simulink model "SustituirTerminoIEnC3"  (R2023a)
settings: Solver=FixedStepDiscrete  StartTime=0.0  StopTime=7430  FixedStep=Delta  RelTol=1e-3
values from neighbouring files (symbols this model uses):
  C2Ini = 1.6    [MassTransferModelData.m]
  C3Ini = 0    [MassTransferModelData.m]
  C4Ini = 0    [MassTransferModelData.m]
  C5Ini = 1.6    [MassTransferModelData.m]
  Delta = 5    [MassTransferModelData.m]
  F = 96485    [MassTransferModelData.m]
  NCells = 120    [MassTransferModelData.m]
  VCell = 0.4968    [MassTransferModelData.m]
  VTank = 500    [MassTransferModelData.m]
  z = 1    [MassTransferModelData.m]
undefined symbols (not defined in the file or in its folder): DiscIntNeverNeededParam
settings Model: Creator=801896  LastModifiedBy=801896

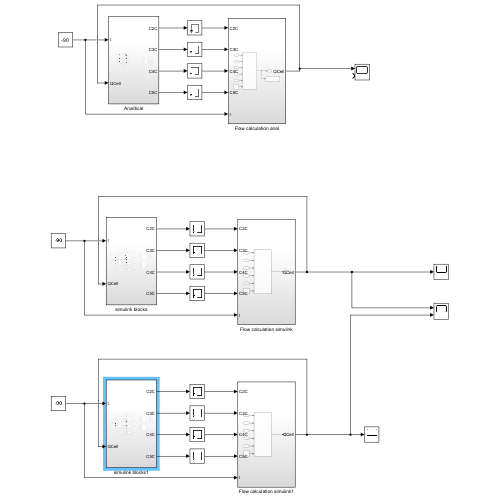
[thumbnail: Simulink's stored preview of the top-level diagram]
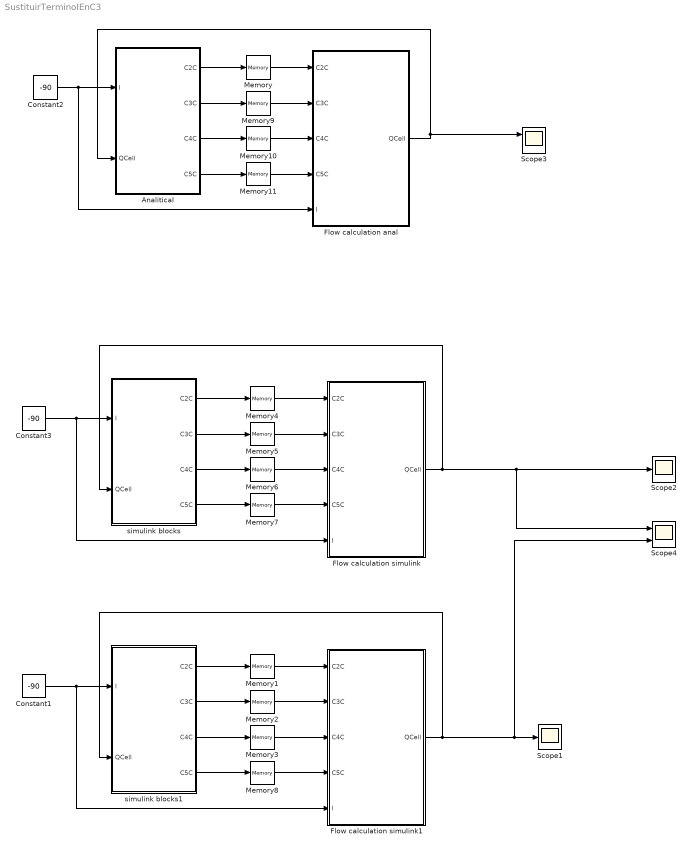
== system SustituirTerminoIEnC3 ==
  Analitical : Subsystem
  Constant1 : Constant  Value=-90
  Constant2 : Constant  Value=-90
  Constant3 : Constant  Value=-90
  Flow calculation anal : Subsystem
  Flow calculation simulink : Subsystem
  Flow calculation simulink1 : Subsystem
  Memory : Memory  InitialCondition=C2Ini
  Memory1 : Memory  InitialCondition=C2Ini
  Memory10 : Memory  InitialCondition=C4Ini
  Memory11 : Memory  InitialCondition=C5Ini
  Memory2 : Memory  InitialCondition=C3Ini
  Memory3 : Memory  InitialCondition=C4Ini
  Memory4 : Memory  InitialCondition=C2Ini
  Memory5 : Memory  InitialCondition=C3Ini
  Memory6 : Memory  InitialCondition=C4Ini
  Memory7 : Memory  InitialCondition=C5Ini
  Memory8 : Memory  InitialCondition=C5Ini
  Memory9 : Memory  InitialCondition=C3Ini
  Scope1 : Scope
  Scope2 : Scope
  Scope3 : Scope  NumInputPorts=2
  Scope4 : Scope  NumInputPorts=2
  simulink blocks : Subsystem
  simulink blocks1 : Subsystem
  wires:
  simulink blocks/3(C4C) -> Memory6/1
  Constant3/1 -> Flow calculation simulink/5(I), simulink blocks/1(I)
  Memory4/1 -> Flow calculation simulink/1(C2C)
  simulink blocks/1(C2C) -> Memory4/1
  Memory6/1 -> Flow calculation simulink/3(C4C)
  Memory7/1 -> Flow calculation simulink/4(C5C)
  simulink blocks/2(C3C) -> Memory5/1
  Memory5/1 -> Flow calculation simulink/2(C3C)
  simulink blocks/4(C5C) -> Memory7/1
  Flow calculation simulink/1(QCell) -> Scope4/1, Scope2/1, simulink blocks/2(QCell)
  Flow calculation simulink1/1(QCell) -> simulink blocks1/2(QCell), Scope4/2, Scope1/1
  simulink blocks1/4(C5C) -> Memory8/1
  Memory2/1 -> Flow calculation simulink1/2(C3C)
  simulink blocks1/2(C3C) -> Memory2/1
  Memory8/1 -> Flow calculation simulink1/4(C5C)
  Memory3/1 -> Flow calculation simulink1/3(C4C)
  simulink blocks1/1(C2C) -> Memory1/1
  Memory1/1 -> Flow calculation simulink1/1(C2C)
  Constant1/1 -> simulink blocks1/1(I), Flow calculation simulink1/5(I)
  simulink blocks1/3(C4C) -> Memory3/1
  Memory/1 -> Flow calculation anal/1(C2C)
  Analitical/1(C2C) -> Memory/1
  Analitical/4(C5C) -> Memory11/1
  Memory9/1 -> Flow calculation anal/2(C3C)
  Memory10/1 -> Flow calculation anal/3(C4C)
  Analitical/3(C4C) -> Memory10/1
  Memory11/1 -> Flow calculation anal/4(C5C)
  Analitical/2(C3C) -> Memory9/1
  Constant2/1 -> Flow calculation anal/5(I), Analitical/1(I)
  Flow calculation anal/1(QCell) -> Analitical/2(QCell), Scope3/1

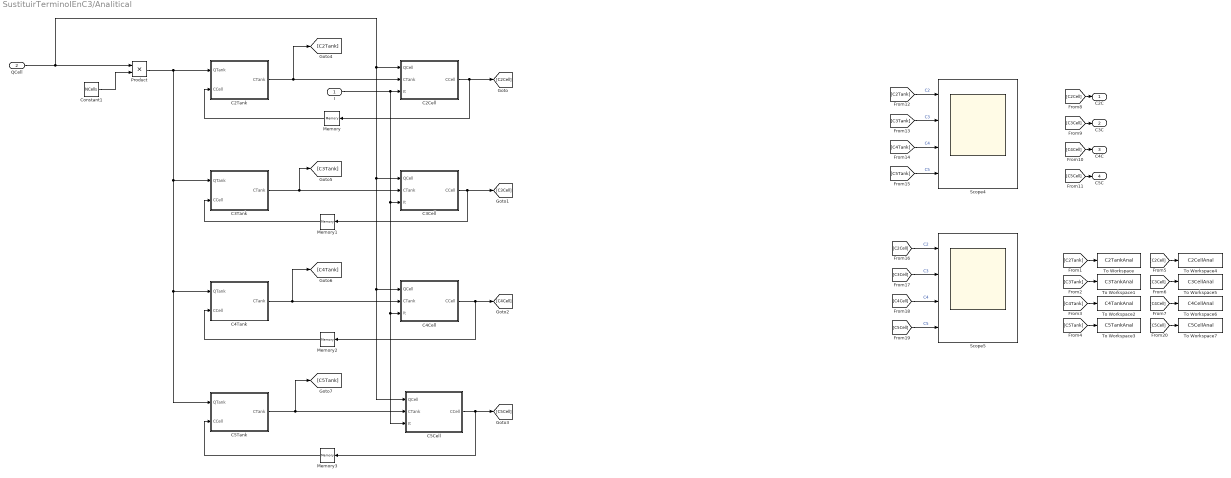
== system SustituirTerminoIEnC3/Analitical ==
  I : Inport
  QCell : Inport  Port=2
  C2Cell : Subsystem
  C2Tank : Subsystem
  C3Cell : Subsystem
  C3Tank : Subsystem
  C4Cell : Subsystem
  C4Tank : Subsystem
  C5Cell : Subsystem
  C5Tank : Subsystem
  Constant1 : Constant  Value=NCells
  Memory : Memory  InitialCondition=C2Ini
  Memory1 : Memory  InitialCondition=C3Ini
  Memory2 : Memory  InitialCondition=C4Ini
  Memory3 : Memory  InitialCondition=C5Ini
  Product : Product
  Scope4 : Scope  NumInputPorts=4
  Scope5 : Scope  NumInputPorts=4
  To Workspace : ToWorkspace  VariableName=C2TankAnal  SaveFormat=Timeseries  SampleTime=-1
  To Workspace1 : ToWorkspace  VariableName=C3TankAnal  SaveFormat=Timeseries  SampleTime=-1
  To Workspace2 : ToWorkspace  VariableName=C4TankAnal  SaveFormat=Timeseries  SampleTime=-1
  To Workspace3 : ToWorkspace  VariableName=C5TankAnal  SaveFormat=Timeseries  SampleTime=-1
  To Workspace4 : ToWorkspace  VariableName=C2CellAnal  SaveFormat=Timeseries  SampleTime=-1
  To Workspace5 : ToWorkspace  VariableName=C3CellAnal  SaveFormat=Timeseries  SampleTime=-1
  To Workspace6 : ToWorkspace  VariableName=C4CellAnal  SaveFormat=Timeseries  SampleTime=-1
  To Workspace7 : ToWorkspace  VariableName=C5CellAnal  SaveFormat=Timeseries  SampleTime=-1
  C2C : Outport
  C3C : Outport  Port=2
  C4C : Outport  Port=3
  C5C : Outport  Port=4
  wires:
  [C5Cell] -> C5C/1
  [C3Cell] -> C3C/1
  [C2Cell] -> C2C/1
  [C4Cell] -> C4C/1
  Constant1/1 -> Product/2
  QCell/1 -> C5Cell/1(QCell), C4Cell/1(QCell), C3Cell/1(QCell), C2Cell/1(QCell), Product/1
  C2Tank/1(CTank) -> [C2Tank], C2Cell/2(CTank)
  C2Cell/1(CCell) -> Memory/1, [C2Cell]
  C3Tank/1(CTank) -> [C3Tank], C3Cell/2(CTank)
  C3Cell/1(CCell) -> Memory1/1, [C3Cell]
  C5Tank/1(CTank) -> [C5Tank], C5Cell/2(CTank)
  C5Cell/1(CCell) -> Memory3/1, [C5Cell]
  C4Cell/1(CCell) -> Memory2/1, [C4Cell]
  C4Tank/1(CTank) -> [C4Tank], C4Cell/2(CTank)
  Product/1 -> C5Tank/1(QTank), C4Tank/1(QTank), C3Tank/1(QTank), C2Tank/1(QTank)
  I/1 -> C3Cell/3(It), C4Cell/3(It), C5Cell/3(It), C2Cell/3(It)
  Memory/1 -> C2Tank/2(CCell)
  Memory1/1 -> C3Tank/2(CCell)
  Memory2/1 -> C4Tank/2(CCell)
  Memory3/1 -> C5Tank/2(CCell)
  [C2Tank] -> Scope4/1  "C2"
  [C3Tank] -> Scope4/2  "C3"
  [C4Tank] -> Scope4/3  "C4"
  [C5Tank] -> Scope4/4  "C5"
  [C2Cell] -> Scope5/1  "C2"
  [C3Cell] -> Scope5/2  "C3"
  [C4Cell] -> Scope5/3  "C4"
  [C5Cell] -> Scope5/4  "C5"
  [C2Tank] -> To Workspace/1
  [C3Tank] -> To Workspace1/1
  [C4Tank] -> To Workspace2/1
  [C5Tank] -> To Workspace3/1
  [C2Cell] -> To Workspace4/1
  [C3Cell] -> To Workspace5/1
  [C4Cell] -> To Workspace6/1
  [C5Cell] -> To Workspace7/1

== system SustituirTerminoIEnC3/Flow calculation anal ==
  C2C : Inport
  C3C : Inport  Port=2
  C4C : Inport  Port=3
  C5C : Inport  Port=4
  I : Inport  Port=5
  Constant : Constant  Value=F
  MATLAB Function : MATLAB Function  TreatAsAtomicUnit=on
  To Workspace : ToWorkspace  VariableName=QCellAnal  SaveFormat=Timeseries  SampleTime=-1
  QCell : Outport
  wires:
  I/1 -> MATLAB Function/5(I)
  Constant/1 -> MATLAB Function/6(F)
  MATLAB Function/1(QCell) -> To Workspace/1, QCell/1
  C2C/1 -> MATLAB Function/1(C2)
  C3C/1 -> MATLAB Function/2(C3)
  C4C/1 -> MATLAB Function/3(C4)
  C5C/1 -> MATLAB Function/4(C5)

== system SustituirTerminoIEnC3/Flow calculation simulink ==
  C2C : Inport
  C3C : Inport  Port=2
  C4C : Inport  Port=3
  C5C : Inport  Port=4
  I : Inport  Port=5
  Constant : Constant  Value=F
  MATLAB Function : MATLAB Function  TreatAsAtomicUnit=on
  QCell : Outport
  wires:
  C5C/1 -> MATLAB Function/4(C5)
  C4C/1 -> MATLAB Function/3(C4)
  C3C/1 -> MATLAB Function/2(C3)
  C2C/1 -> MATLAB Function/1(C2)
  MATLAB Function/1(QCell) -> QCell/1
  Constant/1 -> MATLAB Function/6(F)
  I/1 -> MATLAB Function/5(I)

== system SustituirTerminoIEnC3/Flow calculation simulink1 ==
  C2C : Inport
  C3C : Inport  Port=2
  C4C : Inport  Port=3
  C5C : Inport  Port=4
  I : Inport  Port=5
  Constant : Constant  Value=F
  MATLAB Function : MATLAB Function  TreatAsAtomicUnit=on
  QCell : Outport
  wires:
  I/1 -> MATLAB Function/5(I)
  Constant/1 -> MATLAB Function/6(F)
  MATLAB Function/1(QCell) -> QCell/1
  C2C/1 -> MATLAB Function/1(C2)
  C3C/1 -> MATLAB Function/2(C3)
  C4C/1 -> MATLAB Function/3(C4)
  C5C/1 -> MATLAB Function/4(C5)

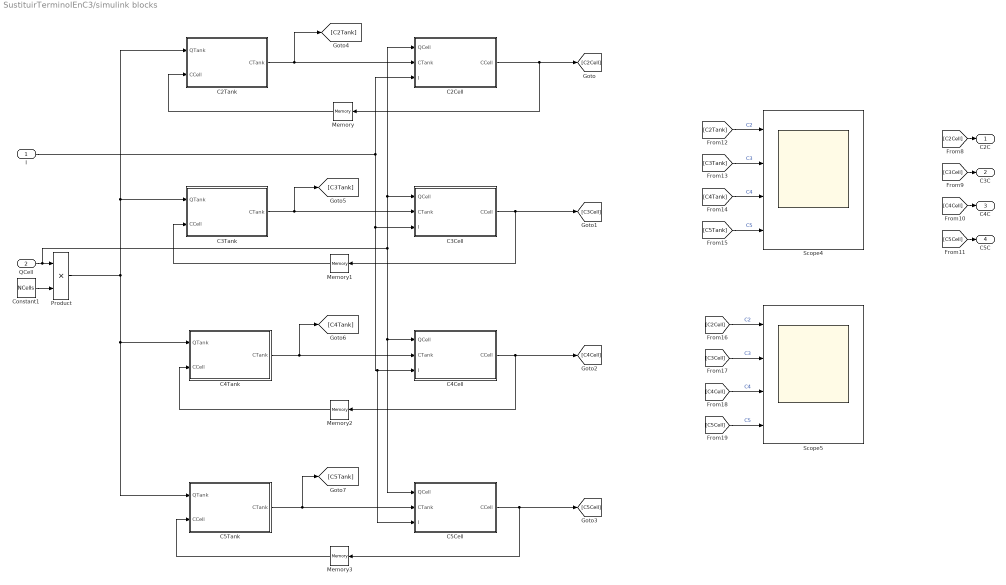
== system SustituirTerminoIEnC3/simulink blocks ==
  I : Inport
  QCell : Inport  Port=2
  C2Cell : Subsystem
  C2Tank : Subsystem
  C3Cell : Subsystem
  C3Tank : Subsystem
  C4Cell : Subsystem
  C4Tank : Subsystem
  C5Cell : Subsystem
  C5Tank : Subsystem
  Constant1 : Constant  Value=NCells
  Memory : Memory  InitialCondition=C2Ini
  Memory1 : Memory  InitialCondition=C3Ini
  Memory2 : Memory  InitialCondition=C4Ini
  Memory3 : Memory  InitialCondition=C5Ini
  Product : Product
  Scope4 : Scope  NumInputPorts=4
  Scope5 : Scope  NumInputPorts=4
  C2C : Outport
  C3C : Outport  Port=2
  C4C : Outport  Port=3
  C5C : Outport  Port=4
  wires:
  Constant1/1 -> Product/2
  QCell/1 -> C2Cell/1(QCell), C3Cell/1(QCell), C5Cell/1(QCell), C4Cell/1(QCell), Product/1
  [C2Cell] -> C2C/1
  [C3Cell] -> C3C/1
  [C4Cell] -> C4C/1
  [C5Cell] -> C5C/1
  C5Tank/1(CTank) -> C5Cell/2(CTank), [C5Tank]
  C4Tank/1(CTank) -> [C4Tank], C4Cell/2(CTank)
  C3Tank/1(CTank) -> [C3Tank], C3Cell/2(CTank)
  C2Tank/1(CTank) -> [C2Tank], C2Cell/2(CTank)
  C2Cell/1(CCell) -> Memory/1, [C2Cell]
  C3Cell/1(CCell) -> [C3Cell], Memory1/1
  C4Cell/1(CCell) -> [C4Cell], Memory2/1
  C5Cell/1(CCell) -> [C5Cell], Memory3/1
  Memory1/1 -> C3Tank/2(CCell)
  Memory2/1 -> C4Tank/2(CCell)
  Memory3/1 -> C5Tank/2(CCell)
  Memory/1 -> C2Tank/2(CCell)
  Product/1 -> C4Tank/1(QTank), C5Tank/1(QTank), C3Tank/1(QTank), C2Tank/1(QTank)
  I/1 -> C2Cell/3(I), C5Cell/3(I), C4Cell/3(I), C3Cell/3(I)
  [C3Tank] -> Scope4/2  "C3"
  [C2Cell] -> Scope5/1  "C2"
  [C4Cell] -> Scope5/3  "C4"
  [C4Tank] -> Scope4/3  "C4"
  [C5Cell] -> Scope5/4  "C5"
  [C3Cell] -> Scope5/2  "C3"
  [C5Tank] -> Scope4/4  "C5"
  [C2Tank] -> Scope4/1  "C2"

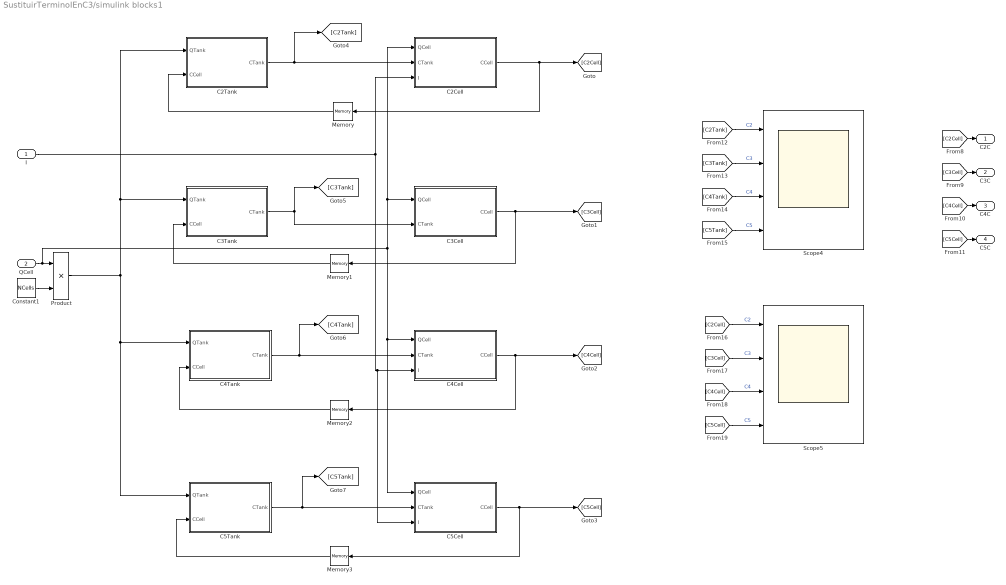
== system SustituirTerminoIEnC3/simulink blocks1 ==
  I : Inport
  QCell : Inport  Port=2
  C2Cell : Subsystem
  C2Tank : Subsystem
  C3Cell : Subsystem
  C3Tank : Subsystem
  C4Cell : Subsystem
  C4Tank : Subsystem
  C5Cell : Subsystem
  C5Tank : Subsystem
  Constant1 : Constant  Value=NCells
  Memory : Memory  InitialCondition=C2Ini
  Memory1 : Memory  InitialCondition=C3Ini
  Memory2 : Memory  InitialCondition=C4Ini
  Memory3 : Memory  InitialCondition=C5Ini
  Product : Product
  Scope4 : Scope  NumInputPorts=4
  Scope5 : Scope  NumInputPorts=4
  C2C : Outport
  C3C : Outport  Port=2
  C4C : Outport  Port=3
  C5C : Outport  Port=4
  wires:
  [C2Tank] -> Scope4/1  "C2"
  [C5Tank] -> Scope4/4  "C5"
  [C3Cell] -> Scope5/2  "C3"
  [C5Cell] -> Scope5/4  "C5"
  [C4Tank] -> Scope4/3  "C4"
  [C4Cell] -> Scope5/3  "C4"
  [C2Cell] -> Scope5/1  "C2"
  [C3Tank] -> Scope4/2  "C3"
  I/1 -> C4Cell/3(I), C5Cell/3(I), C2Cell/3(I)
  Product/1 -> C2Tank/1(QTank), C3Tank/1(QTank), C5Tank/1(QTank), C4Tank/1(QTank)
  Memory/1 -> C2Tank/2(CCell)
  Memory3/1 -> C5Tank/2(CCell)
  Memory2/1 -> C4Tank/2(CCell)
  Memory1/1 -> C3Tank/2(CCell)
  C5Cell/1(CCell) -> Memory3/1, [C5Cell]
  C4Cell/1(CCell) -> Memory2/1, [C4Cell]
  C3Cell/1(CCell) -> Memory1/1, [C3Cell]
  C2Cell/1(CCell) -> [C2Cell], Memory/1
  C2Tank/1(CTank) -> C2Cell/2(CTank), [C2Tank]
  C3Tank/1(CTank) -> C3Cell/2(CTank), [C3Tank]
  C4Tank/1(CTank) -> C4Cell/2(CTank), [C4Tank]
  C5Tank/1(CTank) -> [C5Tank], C5Cell/2(CTank)
  [C5Cell] -> C5C/1
  [C4Cell] -> C4C/1
  [C3Cell] -> C3C/1
  [C2Cell] -> C2C/1
  QCell/1 -> Product/1, C4Cell/1(QCell), C5Cell/1(QCell), C2Cell/1(QCell), C3Cell/1(QCell)
  Constant1/1 -> Product/2

== system SustituirTerminoIEnC3/Analitical/C2Cell ==
  QCell : Inport
  CTank : Inport  Port=2
  It : Inport  Port=3
  Constant : Constant  Value=-1
  Constant1 : Constant  Value=Delta
  Constant2 : Constant
  Constant3 : Constant  Value=F
  Constant4 : Constant  Value=VCell
  MATLAB Function : MATLAB Function  TreatAsAtomicUnit=on
  Memory : Memory  InitialCondition=C2Ini
  CCell : Outport
  wires:
  Constant/1 -> MATLAB Function/8(Sign)
  Constant1/1 -> MATLAB Function/9(Delta)
  Constant2/1 -> MATLAB Function/7(Z)
  QCell/1 -> MATLAB Function/1(QCell)
  Constant3/1 -> MATLAB Function/6(F)
  Constant4/1 -> MATLAB Function/4(VCell)
  MATLAB Function/1(CCell) -> Memory/1, CCell/1
  Memory/1 -> MATLAB Function/3(CCellAnt)
  It/1 -> MATLAB Function/5(It)
  CTank/1 -> MATLAB Function/2(CTank)

== system SustituirTerminoIEnC3/Analitical/C2Tank ==
  QTank : Inport
  CCell : Inport  Port=2
  Constant : Constant  Value=Delta
  Constant1 : Constant  Value=VTank
  MATLAB Function : MATLAB Function  TreatAsAtomicUnit=on
  Memory : Memory  InitialCondition=C2Ini
  Scope4 : Scope
  CTank : Outport
  wires:
  Constant/1 -> MATLAB Function/5(Delta)
  Constant1/1 -> MATLAB Function/4(VTank)
  MATLAB Function/1(CTank) -> Memory/1, CTank/1
  Memory/1 -> MATLAB Function/3(CTankAnt)
  QTank/1 -> MATLAB Function/1(Q)
  CCell/1 -> Scope4/1, MATLAB Function/2(CCell)

== system SustituirTerminoIEnC3/Analitical/C3Cell ==
  QCell : Inport
  CTank : Inport  Port=2
  It : Inport  Port=3
  Constant : Constant
  Constant1 : Constant  Value=Delta
  Constant2 : Constant
  Constant3 : Constant  Value=F
  Constant4 : Constant  Value=VCell
  MATLAB Function : MATLAB Function  TreatAsAtomicUnit=on
  Memory : Memory  InitialCondition=C3Ini
  CCell : Outport
  wires:
  It/1 -> MATLAB Function/5(It)
  Memory/1 -> MATLAB Function/3(CCellAnt)
  MATLAB Function/1(CCell) -> Memory/1, CCell/1
  Constant4/1 -> MATLAB Function/4(VCell)
  Constant3/1 -> MATLAB Function/6(F)
  QCell/1 -> MATLAB Function/1(QCell)
  Constant2/1 -> MATLAB Function/7(Z)
  Constant1/1 -> MATLAB Function/9(Delta)
  Constant/1 -> MATLAB Function/8(Sign)
  CTank/1 -> MATLAB Function/2(CTank)

== system SustituirTerminoIEnC3/Analitical/C3Tank ==
  QTank : Inport
  CCell : Inport  Port=2
  Constant : Constant  Value=Delta
  Constant1 : Constant  Value=VTank
  MATLAB Function : MATLAB Function  TreatAsAtomicUnit=on
  Memory : Memory  InitialCondition=C3Ini
  CTank : Outport
  wires:
  QTank/1 -> MATLAB Function/1(Q)
  Memory/1 -> MATLAB Function/3(CTankAnt)
  MATLAB Function/1(CTank) -> Memory/1, CTank/1
  Constant1/1 -> MATLAB Function/4(VTank)
  Constant/1 -> MATLAB Function/5(Delta)
  CCell/1 -> MATLAB Function/2(CCell)

== system SustituirTerminoIEnC3/Analitical/C4Cell ==
  QCell : Inport
  CTank : Inport  Port=2
  It : Inport  Port=3
  Constant : Constant
  Constant1 : Constant  Value=Delta
  Constant2 : Constant
  Constant3 : Constant  Value=F
  Constant4 : Constant  Value=VCell
  MATLAB Function : MATLAB Function  TreatAsAtomicUnit=on
  Memory : Memory  InitialCondition=C4Ini
  CCell : Outport
  wires:
  Constant/1 -> MATLAB Function/8(Sign)
  Constant1/1 -> MATLAB Function/9(Delta)
  Constant2/1 -> MATLAB Function/7(Z)
  QCell/1 -> MATLAB Function/1(QCell)
  Constant3/1 -> MATLAB Function/6(F)
  Constant4/1 -> MATLAB Function/4(VCell)
  MATLAB Function/1(CCell) -> Memory/1, CCell/1
  Memory/1 -> MATLAB Function/3(CCellAnt)
  It/1 -> MATLAB Function/5(It)
  CTank/1 -> MATLAB Function/2(CTank)

== system SustituirTerminoIEnC3/Analitical/C4Tank ==
  QTank : Inport
  CCell : Inport  Port=2
  Constant : Constant  Value=Delta
  Constant1 : Constant  Value=VTank
  MATLAB Function : MATLAB Function  TreatAsAtomicUnit=on
  Memory : Memory  InitialCondition=C4Ini
  CTank : Outport
  wires:
  Constant/1 -> MATLAB Function/5(Delta)
  Constant1/1 -> MATLAB Function/4(VTank)
  MATLAB Function/1(CTank) -> Memory/1, CTank/1
  Memory/1 -> MATLAB Function/3(CTankAnt)
  QTank/1 -> MATLAB Function/1(Q)
  CCell/1 -> MATLAB Function/2(CCell)

== system SustituirTerminoIEnC3/Analitical/C5Cell ==
  QCell : Inport
  CTank : Inport  Port=2
  It : Inport  Port=3
  Constant : Constant  Value=-1
  Constant1 : Constant  Value=Delta
  Constant2 : Constant
  Constant3 : Constant  Value=F
  Constant4 : Constant  Value=VCell
  MATLAB Function : MATLAB Function  TreatAsAtomicUnit=on
  Memory : Memory  InitialCondition=C5Ini
  CCell : Outport
  wires:
  It/1 -> MATLAB Function/5(It)
  Memory/1 -> MATLAB Function/3(CCellAnt)
  MATLAB Function/1(CCell) -> Memory/1, CCell/1
  Constant4/1 -> MATLAB Function/4(VCell)
  Constant3/1 -> MATLAB Function/6(F)
  QCell/1 -> MATLAB Function/1(QCell)
  Constant2/1 -> MATLAB Function/7(Z)
  Constant1/1 -> MATLAB Function/9(Delta)
  Constant/1 -> MATLAB Function/8(Sign)
  CTank/1 -> MATLAB Function/2(CTank)

== system SustituirTerminoIEnC3/Analitical/C5Tank ==
  QTank : Inport
  CCell : Inport  Port=2
  Constant : Constant  Value=Delta
  Constant1 : Constant  Value=VTank
  MATLAB Function : MATLAB Function  TreatAsAtomicUnit=on
  Memory : Memory  InitialCondition=C5Ini
  Scope : Scope
  CTank : Outport
  wires:
  QTank/1 -> MATLAB Function/1(Q)
  Memory/1 -> MATLAB Function/3(CTankAnt)
  MATLAB Function/1(CTank) -> Memory/1, CTank/1
  Constant1/1 -> MATLAB Function/4(VTank)
  Constant/1 -> MATLAB Function/5(Delta)
  CCell/1 -> MATLAB Function/2(CCell), Scope/1

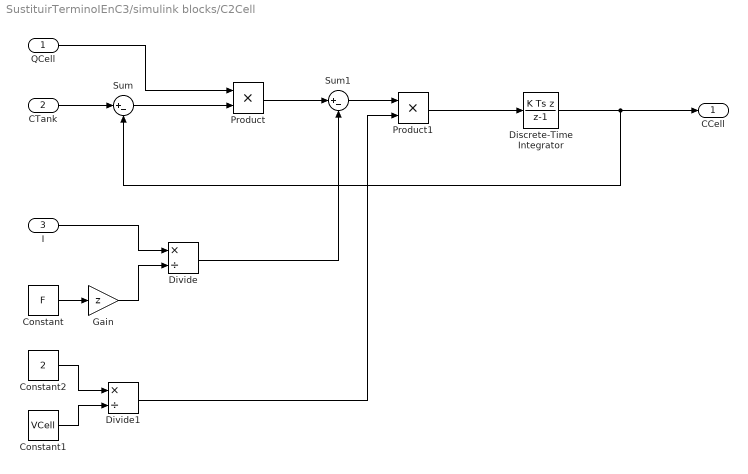
== system SustituirTerminoIEnC3/simulink blocks/C2Cell ==
  QCell : Inport
  CTank : Inport  Port=2
  I : Inport  Port=3
  Constant : Constant  Value=F
  Constant1 : Constant  Value=VCell
  Constant2 : Constant  Value=2
  Discrete-Time Integrator : DiscreteIntegrator  IntegratorMethod=Integration: Backward Euler  InitialCondition=C2Ini  SampleTime=-1  ICPrevOutput=DiscIntNeverNeededParam  ICPrevScaledInput=DiscIntNeverNeededParam
  Divide : Product  Inputs=*/
  Divide1 : Product  Inputs=*/
  Gain : Gain  Gain=z
  Product : Product
  Product1 : Product
  Sum : Sum  Inputs=|+-
  Sum1 : Sum  Inputs=|+-
  CCell : Outport
  wires:
  I/1 -> Divide/1
  Constant/1 -> Gain/1
  Gain/1 -> Divide/2
  Constant1/1 -> Divide1/2
  Constant2/1 -> Divide1/1
  CTank/1 -> Sum/1
  Sum/1 -> Product/2
  QCell/1 -> Product/1
  Product/1 -> Sum1/1
  Divide/1 -> Sum1/2
  Sum1/1 -> Product1/1
  Divide1/1 -> Product1/2
  Product1/1 -> Discrete-Time Integrator/1
  Discrete-Time Integrator/1 -> Sum/2, CCell/1

== system SustituirTerminoIEnC3/simulink blocks/C2Tank ==
  QTank : Inport
  CCell : Inport  Port=2
  Constant : Constant  Value=VTank
  Discrete-Time Integrator : DiscreteIntegrator  IntegratorMethod=Integration: Backward Euler  InitialCondition=C2Ini  SampleTime=-1  ICPrevOutput=DiscIntNeverNeededParam  ICPrevScaledInput=DiscIntNeverNeededParam
  Divide : Product  Inputs=*/
  Product : Product
  Scope4 : Scope
  Sum : Sum  Inputs=|+-
  CTank : Outport
  wires:
  CCell/1 -> Sum/1, Scope4/1
  Sum/1 -> Product/1
  QTank/1 -> Divide/1
  Constant/1 -> Divide/2
  Divide/1 -> Product/2
  Product/1 -> Discrete-Time Integrator/1
  Discrete-Time Integrator/1 -> Sum/2, CTank/1

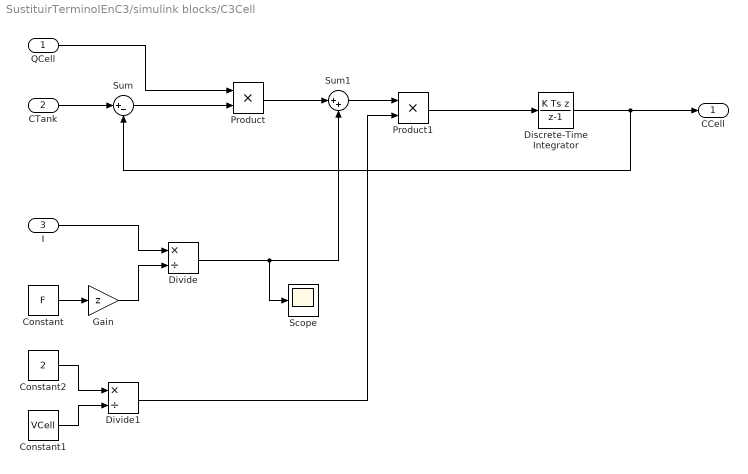
== system SustituirTerminoIEnC3/simulink blocks/C3Cell ==
  QCell : Inport
  CTank : Inport  Port=2
  I : Inport  Port=3
  Constant : Constant  Value=F
  Constant1 : Constant  Value=VCell
  Constant2 : Constant  Value=2
  Discrete-Time Integrator : DiscreteIntegrator  IntegratorMethod=Integration: Backward Euler  InitialCondition=C3Ini  SampleTime=-1  ICPrevOutput=DiscIntNeverNeededParam  ICPrevScaledInput=DiscIntNeverNeededParam
  Divide : Product  Inputs=*/
  Divide1 : Product  Inputs=*/
  Gain : Gain  Gain=z
  Product : Product
  Product1 : Product
  Scope : Scope
  Sum : Sum  Inputs=|+-
  Sum1 : Sum  Inputs=|++
  CCell : Outport
  wires:
  Product1/1 -> Discrete-Time Integrator/1
  Divide1/1 -> Product1/2
  Sum1/1 -> Product1/1
  Divide/1 -> Scope/1, Sum1/2
  Product/1 -> Sum1/1
  QCell/1 -> Product/1
  Sum/1 -> Product/2
  CTank/1 -> Sum/1
  Constant2/1 -> Divide1/1
  Constant1/1 -> Divide1/2
  Gain/1 -> Divide/2
  Constant/1 -> Gain/1
  I/1 -> Divide/1
  Discrete-Time Integrator/1 -> Sum/2, CCell/1

== system SustituirTerminoIEnC3/simulink blocks/C3Tank ==
  QTank : Inport
  CCell : Inport  Port=2
  Constant : Constant  Value=VTank
  Discrete-Time Integrator : DiscreteIntegrator  IntegratorMethod=Integration: Backward Euler  InitialCondition=C3Ini  SampleTime=-1  ICPrevOutput=DiscIntNeverNeededParam  ICPrevScaledInput=DiscIntNeverNeededParam
  Divide : Product  Inputs=*/
  Product : Product
  Sum : Sum  Inputs=|+-
  CTank : Outport
  wires:
  Product/1 -> Discrete-Time Integrator/1
  Divide/1 -> Product/2
  Constant/1 -> Divide/2
  QTank/1 -> Divide/1
  Sum/1 -> Product/1
  CCell/1 -> Sum/1
  Discrete-Time Integrator/1 -> Sum/2, CTank/1

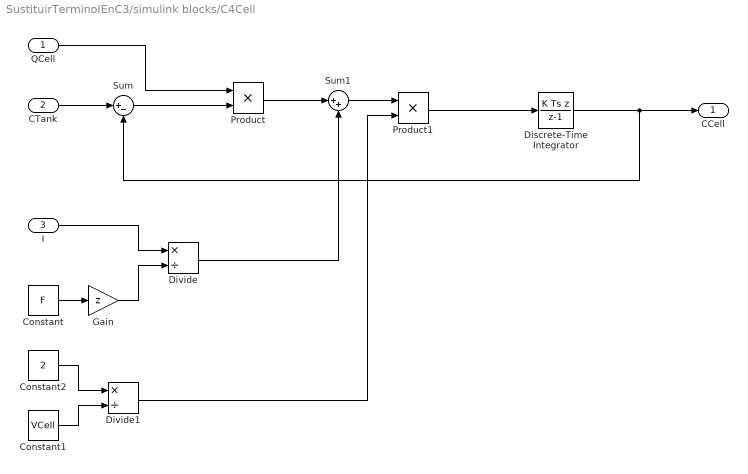
== system SustituirTerminoIEnC3/simulink blocks/C4Cell ==
  QCell : Inport
  CTank : Inport  Port=2
  I : Inport  Port=3
  Constant : Constant  Value=F
  Constant1 : Constant  Value=VCell
  Constant2 : Constant  Value=2
  Discrete-Time Integrator : DiscreteIntegrator  IntegratorMethod=Integration: Backward Euler  InitialCondition=C4Ini  SampleTime=-1  ICPrevOutput=DiscIntNeverNeededParam  ICPrevScaledInput=DiscIntNeverNeededParam
  Divide : Product  Inputs=*/
  Divide1 : Product  Inputs=*/
  Gain : Gain  Gain=z
  Product : Product
  Product1 : Product
  Sum : Sum  Inputs=|+-
  Sum1 : Sum  Inputs=|++
  CCell : Outport
  wires:
  I/1 -> Divide/1
  Constant/1 -> Gain/1
  Gain/1 -> Divide/2
  Constant1/1 -> Divide1/2
  Constant2/1 -> Divide1/1
  CTank/1 -> Sum/1
  Sum/1 -> Product/2
  QCell/1 -> Product/1
  Product/1 -> Sum1/1
  Divide/1 -> Sum1/2
  Sum1/1 -> Product1/1
  Divide1/1 -> Product1/2
  Product1/1 -> Discrete-Time Integrator/1
  Discrete-Time Integrator/1 -> Sum/2, CCell/1

== system SustituirTerminoIEnC3/simulink blocks/C4Tank ==
  QTank : Inport
  CCell : Inport  Port=2
  Constant : Constant  Value=VTank
  Discrete-Time Integrator : DiscreteIntegrator  IntegratorMethod=Integration: Backward Euler  InitialCondition=C4Ini  SampleTime=-1  ICPrevOutput=DiscIntNeverNeededParam  ICPrevScaledInput=DiscIntNeverNeededParam
  Divide : Product  Inputs=*/
  Product : Product
  Sum : Sum  Inputs=|+-
  CTank : Outport
  wires:
  CCell/1 -> Sum/1
  Sum/1 -> Product/1
  QTank/1 -> Divide/1
  Constant/1 -> Divide/2
  Divide/1 -> Product/2
  Product/1 -> Discrete-Time Integrator/1
  Discrete-Time Integrator/1 -> Sum/2, CTank/1

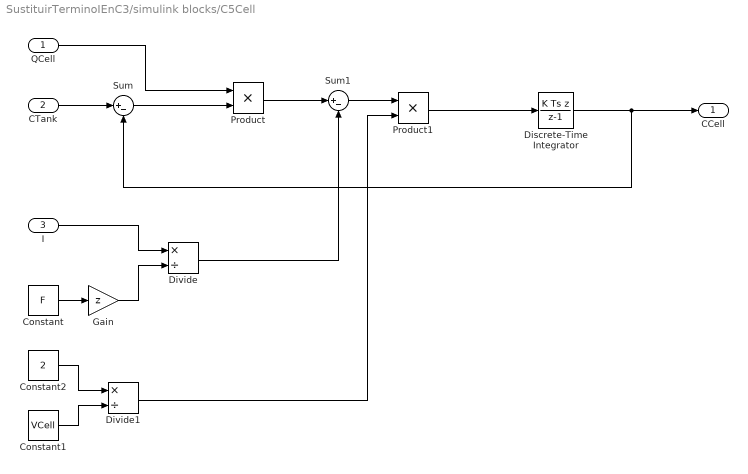
== system SustituirTerminoIEnC3/simulink blocks/C5Cell ==
  QCell : Inport
  CTank : Inport  Port=2
  I : Inport  Port=3
  Constant : Constant  Value=F
  Constant1 : Constant  Value=VCell
  Constant2 : Constant  Value=2
  Discrete-Time Integrator : DiscreteIntegrator  IntegratorMethod=Integration: Backward Euler  InitialCondition=C5Ini  SampleTime=-1  ICPrevOutput=DiscIntNeverNeededParam  ICPrevScaledInput=DiscIntNeverNeededParam
  Divide : Product  Inputs=*/
  Divide1 : Product  Inputs=*/
  Gain : Gain  Gain=z
  Product : Product
  Product1 : Product
  Sum : Sum  Inputs=|+-
  Sum1 : Sum  Inputs=|+-
  CCell : Outport
  wires:
  Product1/1 -> Discrete-Time Integrator/1
  Divide1/1 -> Product1/2
  Sum1/1 -> Product1/1
  Divide/1 -> Sum1/2
  Product/1 -> Sum1/1
  QCell/1 -> Product/1
  Sum/1 -> Product/2
  CTank/1 -> Sum/1
  Constant2/1 -> Divide1/1
  Constant1/1 -> Divide1/2
  Gain/1 -> Divide/2
  Constant/1 -> Gain/1
  I/1 -> Divide/1
  Discrete-Time Integrator/1 -> Sum/2, CCell/1

== system SustituirTerminoIEnC3/simulink blocks/C5Tank ==
  QTank : Inport
  CCell : Inport  Port=2
  Constant : Constant  Value=VTank
  Discrete-Time Integrator : DiscreteIntegrator  IntegratorMethod=Integration: Backward Euler  InitialCondition=C5Ini  SampleTime=-1  ICPrevOutput=DiscIntNeverNeededParam  ICPrevScaledInput=DiscIntNeverNeededParam
  Divide : Product  Inputs=*/
  Product : Product
  Sum : Sum  Inputs=|+-
  CTank : Outport
  wires:
  Product/1 -> Discrete-Time Integrator/1
  Divide/1 -> Product/2
  Constant/1 -> Divide/2
  QTank/1 -> Divide/1
  Sum/1 -> Product/1
  CCell/1 -> Sum/1
  Discrete-Time Integrator/1 -> Sum/2, CTank/1

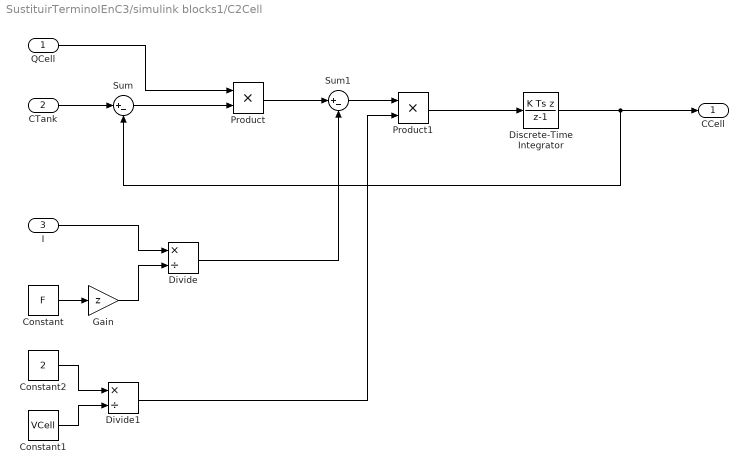
== system SustituirTerminoIEnC3/simulink blocks1/C2Cell ==
  QCell : Inport
  CTank : Inport  Port=2
  I : Inport  Port=3
  Constant : Constant  Value=F
  Constant1 : Constant  Value=VCell
  Constant2 : Constant  Value=2
  Discrete-Time Integrator : DiscreteIntegrator  IntegratorMethod=Integration: Backward Euler  InitialCondition=C2Ini  SampleTime=-1  ICPrevOutput=DiscIntNeverNeededParam  ICPrevScaledInput=DiscIntNeverNeededParam
  Divide : Product  Inputs=*/
  Divide1 : Product  Inputs=*/
  Gain : Gain  Gain=z
  Product : Product
  Product1 : Product
  Sum : Sum  Inputs=|+-
  Sum1 : Sum  Inputs=|+-
  CCell : Outport
  wires:
  Discrete-Time Integrator/1 -> CCell/1, Sum/2
  Product1/1 -> Discrete-Time Integrator/1
  Divide1/1 -> Product1/2
  Sum1/1 -> Product1/1
  Divide/1 -> Sum1/2
  Product/1 -> Sum1/1
  QCell/1 -> Product/1
  Sum/1 -> Product/2
  CTank/1 -> Sum/1
  Constant2/1 -> Divide1/1
  Constant1/1 -> Divide1/2
  Gain/1 -> Divide/2
  Constant/1 -> Gain/1
  I/1 -> Divide/1

== system SustituirTerminoIEnC3/simulink blocks1/C2Tank ==
  QTank : Inport
  CCell : Inport  Port=2
  Constant : Constant  Value=VTank
  Discrete-Time Integrator : DiscreteIntegrator  IntegratorMethod=Integration: Backward Euler  InitialCondition=C2Ini  SampleTime=-1  ICPrevOutput=DiscIntNeverNeededParam  ICPrevScaledInput=DiscIntNeverNeededParam
  Divide : Product  Inputs=*/
  Product : Product
  Scope4 : Scope
  Sum : Sum  Inputs=|+-
  CTank : Outport
  wires:
  Discrete-Time Integrator/1 -> CTank/1, Sum/2
  Product/1 -> Discrete-Time Integrator/1
  Divide/1 -> Product/2
  Constant/1 -> Divide/2
  QTank/1 -> Divide/1
  Sum/1 -> Product/1
  CCell/1 -> Scope4/1, Sum/1

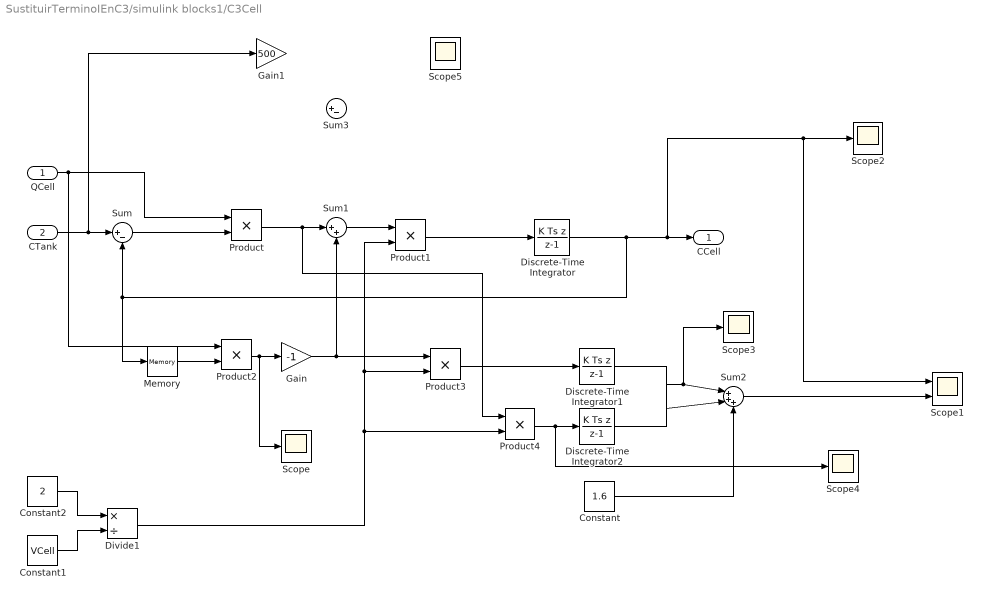
== system SustituirTerminoIEnC3/simulink blocks1/C3Cell ==
  QCell : Inport
  CTank : Inport  Port=2
  Constant : Constant  Value=1.6
  Constant1 : Constant  Value=VCell
  Constant2 : Constant  Value=2
  Discrete-Time Integrator : DiscreteIntegrator  IntegratorMethod=Integration: Backward Euler  InitialCondition=C3Ini  SampleTime=-1  ICPrevOutput=DiscIntNeverNeededParam  ICPrevScaledInput=DiscIntNeverNeededParam
  Discrete-Time Integrator1 : DiscreteIntegrator  IntegratorMethod=Integration: Backward Euler  SampleTime=-1  ICPrevOutput=DiscIntNeverNeededParam  ICPrevScaledInput=DiscIntNeverNeededParam
  Discrete-Time Integrator2 : DiscreteIntegrator  IntegratorMethod=Integration: Backward Euler  SampleTime=-1  ICPrevOutput=DiscIntNeverNeededParam  ICPrevScaledInput=DiscIntNeverNeededParam
  Divide1 : Product  Inputs=*/
  Gain : Gain  Gain=-1
  Gain1 : Gain  Gain=500
  Memory : Memory  InitialCondition=C3Ini
  Product{,1..4} (5 alike) : Product
  Scope{,2..5} (5 alike) : Scope
  Scope1 : Scope  NumInputPorts=2
  Sum : Sum  Inputs=|+-
  Sum1 : Sum  Inputs=|++
  Sum2 : Sum  Inputs=|+++
  Sum3 : Sum  Inputs=|+-
  CCell : Outport
  wires:
  Discrete-Time Integrator/1 -> Scope1/1, Scope2/1, CCell/1, Memory/1, Sum/2
  Constant1/1 -> Divide1/2
  Constant2/1 -> Divide1/1
  CTank/1 -> Gain1/1, Sum/1
  Sum/1 -> Product/2
  QCell/1 -> Product2/1, Product/1
  Product/1 -> Product4/1, Sum1/1
  Sum1/1 -> Product1/1
  Divide1/1 -> Product4/2, Product3/2, Product1/2
  Product1/1 -> Discrete-Time Integrator/1
  Gain/1 -> Sum1/2, Product3/1
  Product2/1 -> Scope/1, Gain/1
  Memory/1 -> Product2/2
  Product3/1 -> Discrete-Time Integrator1/1
  Product4/1 -> Scope4/1, Discrete-Time Integrator2/1
  Discrete-Time Integrator1/1 -> Sum2/2
  Discrete-Time Integrator2/1 -> Scope3/1, Sum2/1
  Sum2/1 -> Scope1/2
  Constant/1 -> Sum2/3

== system SustituirTerminoIEnC3/simulink blocks1/C3Tank ==
  QTank : Inport
  CCell : Inport  Port=2
  Constant : Constant  Value=VTank
  Discrete-Time Integrator : DiscreteIntegrator  IntegratorMethod=Integration: Backward Euler  InitialCondition=C3Ini  SampleTime=-1  ICPrevOutput=DiscIntNeverNeededParam  ICPrevScaledInput=DiscIntNeverNeededParam
  Divide : Product  Inputs=*/
  Product : Product
  Sum : Sum  Inputs=|+-
  CTank : Outport
  wires:
  Discrete-Time Integrator/1 -> CTank/1, Sum/2
  CCell/1 -> Sum/1
  Sum/1 -> Product/1
  QTank/1 -> Divide/1
  Constant/1 -> Divide/2
  Divide/1 -> Product/2
  Product/1 -> Discrete-Time Integrator/1

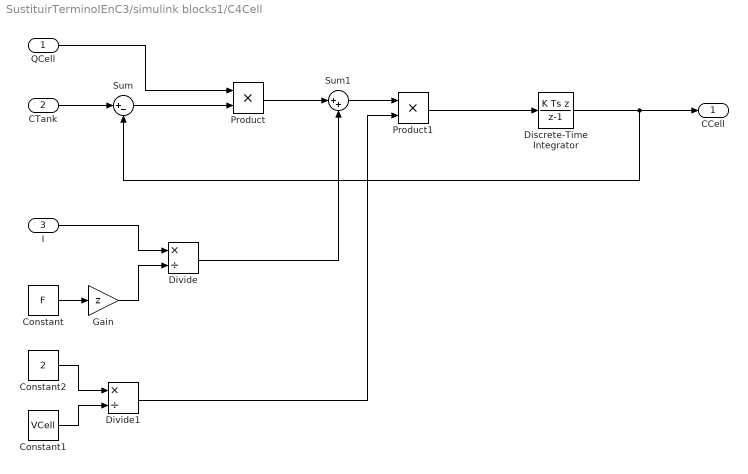
== system SustituirTerminoIEnC3/simulink blocks1/C4Cell ==
  QCell : Inport
  CTank : Inport  Port=2
  I : Inport  Port=3
  Constant : Constant  Value=F
  Constant1 : Constant  Value=VCell
  Constant2 : Constant  Value=2
  Discrete-Time Integrator : DiscreteIntegrator  IntegratorMethod=Integration: Backward Euler  InitialCondition=C4Ini  SampleTime=-1  ICPrevOutput=DiscIntNeverNeededParam  ICPrevScaledInput=DiscIntNeverNeededParam
  Divide : Product  Inputs=*/
  Divide1 : Product  Inputs=*/
  Gain : Gain  Gain=z
  Product : Product
  Product1 : Product
  Sum : Sum  Inputs=|+-
  Sum1 : Sum  Inputs=|++
  CCell : Outport
  wires:
  Discrete-Time Integrator/1 -> CCell/1, Sum/2
  Product1/1 -> Discrete-Time Integrator/1
  Divide1/1 -> Product1/2
  Sum1/1 -> Product1/1
  Divide/1 -> Sum1/2
  Product/1 -> Sum1/1
  QCell/1 -> Product/1
  Sum/1 -> Product/2
  CTank/1 -> Sum/1
  Constant2/1 -> Divide1/1
  Constant1/1 -> Divide1/2
  Gain/1 -> Divide/2
  Constant/1 -> Gain/1
  I/1 -> Divide/1

== system SustituirTerminoIEnC3/simulink blocks1/C4Tank ==
  QTank : Inport
  CCell : Inport  Port=2
  Constant : Constant  Value=VTank
  Discrete-Time Integrator : DiscreteIntegrator  IntegratorMethod=Integration: Backward Euler  InitialCondition=C4Ini  SampleTime=-1  ICPrevOutput=DiscIntNeverNeededParam  ICPrevScaledInput=DiscIntNeverNeededParam
  Divide : Product  Inputs=*/
  Product : Product
  Sum : Sum  Inputs=|+-
  CTank : Outport
  wires:
  Discrete-Time Integrator/1 -> CTank/1, Sum/2
  Product/1 -> Discrete-Time Integrator/1
  Divide/1 -> Product/2
  Constant/1 -> Divide/2
  QTank/1 -> Divide/1
  Sum/1 -> Product/1
  CCell/1 -> Sum/1

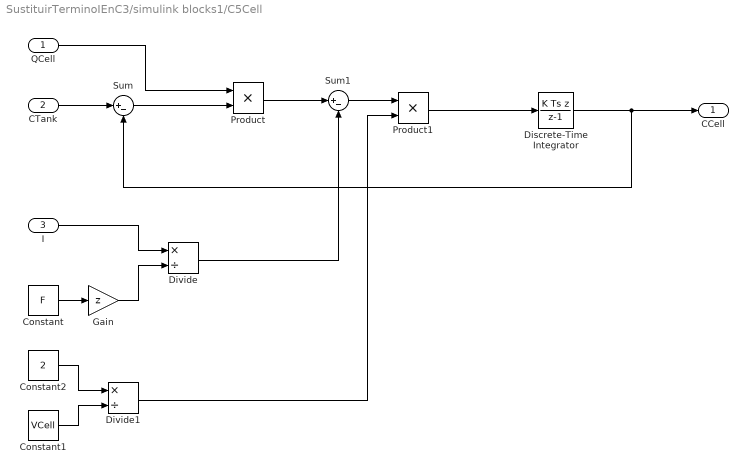
== system SustituirTerminoIEnC3/simulink blocks1/C5Cell ==
  QCell : Inport
  CTank : Inport  Port=2
  I : Inport  Port=3
  Constant : Constant  Value=F
  Constant1 : Constant  Value=VCell
  Constant2 : Constant  Value=2
  Discrete-Time Integrator : DiscreteIntegrator  IntegratorMethod=Integration: Backward Euler  InitialCondition=C5Ini  SampleTime=-1  ICPrevOutput=DiscIntNeverNeededParam  ICPrevScaledInput=DiscIntNeverNeededParam
  Divide : Product  Inputs=*/
  Divide1 : Product  Inputs=*/
  Gain : Gain  Gain=z
  Product : Product
  Product1 : Product
  Sum : Sum  Inputs=|+-
  Sum1 : Sum  Inputs=|+-
  CCell : Outport
  wires:
  Discrete-Time Integrator/1 -> CCell/1, Sum/2
  I/1 -> Divide/1
  Constant/1 -> Gain/1
  Gain/1 -> Divide/2
  Constant1/1 -> Divide1/2
  Constant2/1 -> Divide1/1
  CTank/1 -> Sum/1
  Sum/1 -> Product/2
  QCell/1 -> Product/1
  Product/1 -> Sum1/1
  Divide/1 -> Sum1/2
  Sum1/1 -> Product1/1
  Divide1/1 -> Product1/2
  Product1/1 -> Discrete-Time Integrator/1

== system SustituirTerminoIEnC3/simulink blocks1/C5Tank ==
  QTank : Inport
  CCell : Inport  Port=2
  Constant : Constant  Value=VTank
  Discrete-Time Integrator : DiscreteIntegrator  IntegratorMethod=Integration: Backward Euler  InitialCondition=C5Ini  SampleTime=-1  ICPrevOutput=DiscIntNeverNeededParam  ICPrevScaledInput=DiscIntNeverNeededParam
  Divide : Product  Inputs=*/
  Product : Product
  Sum : Sum  Inputs=|+-
  CTank : Outport
  wires:
  Discrete-Time Integrator/1 -> CTank/1, Sum/2
  CCell/1 -> Sum/1
  Sum/1 -> Product/1
  QTank/1 -> Divide/1
  Constant/1 -> Divide/2
  Divide/1 -> Product/2
  Product/1 -> Discrete-Time Integrator/1

== matlab function SustituirTerminoIEnC3/Analitical/C5Cell/MATLAB Function ==
  data: QCell input; CCell output; CTank input; CCellAnt input; VCell input; It input; F input; Z input; Sign input; Delta input
function CCell = fcn(QCell, CTank, CCellAnt, VCell, It, F, Z, Sign, Delta)
    K1 = QCell*(1/(VCell/2));
    K2 = (1/(VCell/2))*(1/(Z*F));
    CCell = (K1*Delta*CTank + Sign*K2*Delta*It + CCellAnt)/(1+K1*Delta);
end

== matlab function SustituirTerminoIEnC3/Analitical/C5Tank/MATLAB Function ==
  data: Q input; CTank output; CCell input; CTankAnt input; VTank input; Delta input
function CTank = fcn(Q, CCell, CTankAnt, VTank, Delta)
    K3 = Q/VTank;
    CTank = (CCell*K3*Delta + CTankAnt)/(1+K3*Delta);
end

== matlab function SustituirTerminoIEnC3/Flow calculation anal/MATLAB Function ==
  data: C2 input; QCell output; C3 input; C4 input; C5 input; I input; F input
function QCell = fcn(C2, C3, C4, C5, I, F)
    if I > 0
        QCell = abs(I)/(F*(C2+C5)/2);
    else
        QCell = abs(I)/(F*(C3+C4)/2);
    end
end

== matlab function SustituirTerminoIEnC3/Flow calculation simulink/MATLAB Function ==
  data: C2 input; QCell output; C3 input; C4 input; C5 input; I input; F input
function QCell = fcn(C2, C3, C4, C5, I, F)
    if I > 0
        QCell = abs(I)/(F*(C2+C5)/2);
    else
        QCell = abs(I)/(F*(C3+C4)/2);
    end
end

== matlab function SustituirTerminoIEnC3/Flow calculation simulink1/MATLAB Function ==
  data: C2 input; QCell output; C3 input; C4 input; C5 input; I input; F input
function QCell = fcn(C2, C3, C4, C5, I, F)
    if I > 0
        QCell = abs(I)/(F*(C2+C5)/2);
    else
        QCell = abs(I)/(F*(C3+C4)/2);
    end
end

== matlab function SustituirTerminoIEnC3/Analitical/C2Cell/MATLAB Function ==
  data: QCell input; CCell output; CTank input; CCellAnt input; VCell input; It input; F input; Z input; Sign input; Delta input
function CCell = fcn(QCell, CTank, CCellAnt, VCell, It, F, Z, Sign, Delta)
    K1 = QCell*(1/(VCell/2));
    K2 = (1/(VCell/2))*(1/(Z*F));
    CCell = (K1*Delta*CTank + Sign*K2*Delta*It + CCellAnt)/(1+K1*Delta);
end

== matlab function SustituirTerminoIEnC3/Analitical/C2Tank/MATLAB Function ==
  data: Q input; CTank output; CCell input; CTankAnt input; VTank input; Delta input
function CTank = fcn(Q, CCell, CTankAnt, VTank, Delta)
    K3 = Q/VTank;
    CTank = (CCell*K3*Delta + CTankAnt)/(1+K3*Delta);
end

== matlab function SustituirTerminoIEnC3/Analitical/C3Cell/MATLAB Function ==
  data: QCell input; CCell output; CTank input; CCellAnt input; VCell input; It input; F input; Z input; Sign input; Delta input
function CCell = fcn(QCell, CTank, CCellAnt, VCell, It, F, Z, Sign, Delta)
    K1 = QCell*(1/(VCell/2));
    K2 = (1/(VCell/2))*(1/(Z*F));
    CCell = (K1*Delta*CTank + Sign*K2*Delta*It + CCellAnt)/(1+K1*Delta);
end

== matlab function SustituirTerminoIEnC3/Analitical/C3Tank/MATLAB Function ==
  data: Q input; CTank output; CCell input; CTankAnt input; VTank input; Delta input
function CTank = fcn(Q, CCell, CTankAnt, VTank, Delta)
    K3 = Q/VTank;
    CTank = (CCell*K3*Delta + CTankAnt)/(1+K3*Delta);
end

== matlab function SustituirTerminoIEnC3/Analitical/C4Cell/MATLAB Function ==
  data: QCell input; CCell output; CTank input; CCellAnt input; VCell input; It input; F input; Z input; Sign input; Delta input
function CCell = fcn(QCell, CTank, CCellAnt, VCell, It, F, Z, Sign, Delta)
    K1 = QCell*(1/(VCell/2));
    K2 = (1/(VCell/2))*(1/(Z*F));
    CCell = (K1*Delta*CTank + Sign*K2*Delta*It + CCellAnt)/(1+K1*Delta);
end

== matlab function SustituirTerminoIEnC3/Analitical/C4Tank/MATLAB Function ==
  data: Q input; CTank output; CCell input; CTankAnt input; VTank input; Delta input
function CTank = fcn(Q, CCell, CTankAnt, VTank, Delta)
    K3 = Q/VTank;
    CTank = (CCell*K3*Delta + CTankAnt)/(1+K3*Delta);
end
